simulink model "Level_Indicator"  (R2019a)
settings: Solver=VariableStepAuto  StartTime=0.0  StopTime=10.0  RelTol=1e-3
settings Model: Creator=admin  LastModifiedBy=admin

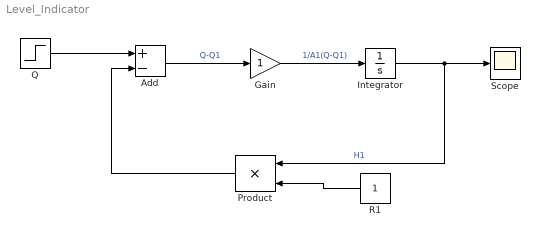
== system Level_Indicator ==
  Add : Sum  Inputs=+-
  Gain : Gain
  Integrator : Integrator
  Product : Product
  Q : Step  SampleTime=0
  "R1 " : Constant
  Scope : Scope
  wires:
  Integrator/1 -> Product/1, Scope/1  "H1"
  Gain/1 -> Integrator/1  "1/A1(Q-Q1)"
  Product/1 -> Add/2
  Q/1 -> Add/1
  "R1 "/1 -> Product/2
  Add/1 -> Gain/1  "Q-Q1"
